simulink model "Simulink_IEEE_39_two_DSR"  (R2021b)
settings: Solver=ode23  StartTime=0.0  StopTime=60  MaxStep=0.2  MinStep=0.0001  RelTol=1e-3  EnableMultiTasking=on
values from neighbouring files (symbols this model uses):
  A = 80    [Monte_Carlo_Simulation.m]
  AC = 0.01    [Monte_Carlo_Simulation.m]
  D = 125    [Monte_Carlo_Simulation.m]
  dP = -300    [Monte_Carlo_Simulation.m]
  FHP = 0.8    [Monte_Carlo_Simulation.m]
  H = 300    [Monte_Carlo_Simulation.m]
  N = 6000/1000    (= 6)    [Monte_Carlo_Simulation.m]
  Pa = DSR_max * rand(1,1)    [Monte_Carlo_Simulation.m]
  Pb = B_max * rand(1,1)    [Monte_Carlo_Simulation.m]
  R = 0.002* ones(gen_num)    [Monte_Carlo_Simulation.m]
  Re = PFR_max .* rand(1,10)    [Monte_Carlo_Simulation.m]
  Ta = 5    [Monte_Carlo_Simulation.m]
  TB = 0.5    [Monte_Carlo_Simulation.m]
  Tc = 0.27    [Monte_Carlo_Simulation.m]
  TCH = 0.6 * ones(10)    [Monte_Carlo_Simulation.m]
  TG = [0.3;0.4;0.5;0.3;0.4;0.5;0.5;0.3;0.4;0.5]*40    [Monte_Carlo_Simulation.m]
  TRH = 5    [Monte_Carlo_Simulation.m]
settings Model: Creator=however  LastModifiedBy=e0546041
settings SolverCC: AlgebraicLoopSolver=TrustRegion
settings DataIOCC: LimitDataPoints=on  SaveFormat=Array  SignalLoggingSaveFormat=ModelDataLogs  ReturnWorkspaceOutputs=off
settings OptimizationCC: ExpressionDepthLimit=2147483647  LifeSpan=inf
settings DebuggingCC: UnderspecifiedInitializationDetection=Classic  MergeDetectMultiDrivingBlocksExec=none  SolverPrmCheckMsg=warning  FcnCallInpInsideContextMsg=warning  StateNameClashWarn=warning  PregeneratedLibrarySubsystemCodeDiagnostic=none  SFUnexpectedBacktrackingDiag=warning  SFNoUnconditionalDefaultTransitionDiag=warning  SFExecutionAtInitializationDiag=none  SFMachineParentedDataDiag=warning  ArithmeticOperatorsInVariantConditions=warning
settings HardwareCC: ProdBitPerPointer=32  ProdBitPerSizeT=32  ProdBitPerPtrDiffT=32  ProdLargestAtomicFloat=None  ProdIntDivRoundTo=Undefined  ProdEndianess=Unspecified  ProdWordSize=32  ProdHWDeviceType=32-bit Generic
settings ModelReferenceCC: PropagateSignalLabelsOutOfModel=off
settings SFSimCC: SimUseLocalCustomCode=off  CustomCodeUndefinedFunction=UseInterfaceOnly
settings RTWCC: RTWUseLocalCustomCode=off
settings CodeAppCC: StateflowObjectComments=on
settings GRTTargetCC: TargetLangStandard=C89/C90 (ANSI)  CombineOutputUpdateFcns=off  GRTInterface=on
settings ConfigComp: CovMetricSettings=dw  CovSaveCumulativeToWorkspaceVar=on  CovSaveSingleToWorkspaceVar=on  CovExternalEMLEnable=off

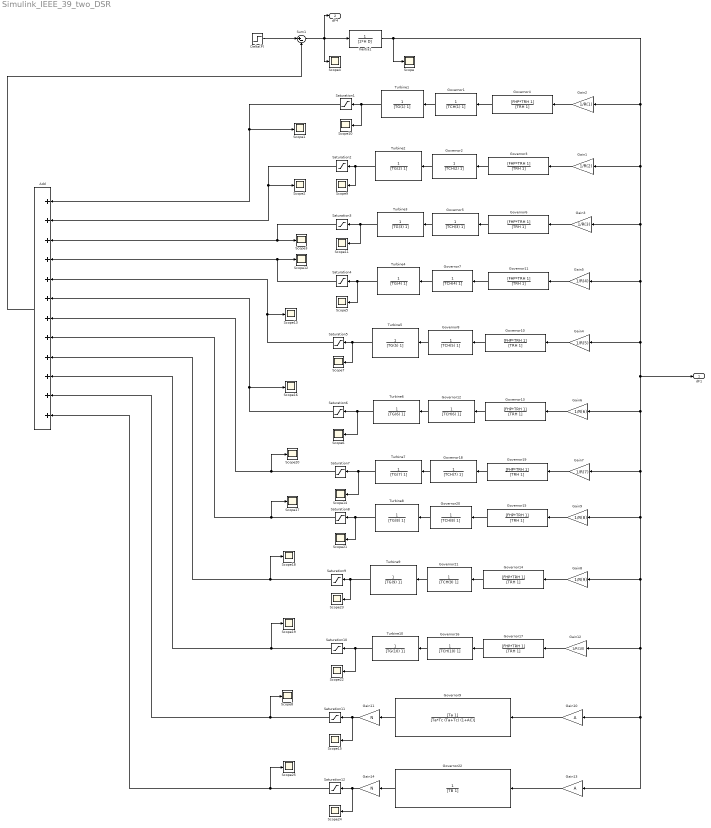
== system Simulink_IEEE_39_two_DSR ==
  Add : Sum  Inputs=++++++++++++
  Delta(P) : Step  Time=0  After=dP  SampleTime=0
  Gain1 : Gain  Gain=1/R(2)
  Gain10 : Gain  Gain=A
  Gain11 : Gain  Gain=N
  Gain12 : Gain  Gain=1/R(10)
  Gain13 : Gain  Gain=A
  Gain14 : Gain  Gain=N
  Gain2 : Gain  Gain=1/R(1)
  Gain3 : Gain  Gain=1/R(3)
  Gain4 : Gain  Gain=1/R(5)
  Gain5 : Gain  Gain=1/R(4)
  Gain6 : Gain  Gain=1/R(6)
  Gain7 : Gain  Gain=1/R(7)
  Gain8 : Gain  Gain=1/R(9)
  Gain9 : Gain  Gain=1/R(8)
  Governor1 : TransferFcn  Denominator=[TCH(1) 1]
  Governor{3..4,6,10..11,13..15,17,19} (10 alike) : TransferFcn  Numerator=[FHP*TRH 1]  Denominator=[TRH 1]
  Governor12 : TransferFcn  Denominator=[TCH(6) 1]
  Governor16 : TransferFcn  Denominator=[TCH(10) 1]
  Governor18 : TransferFcn  Denominator=[TCH(7) 1]
  Governor2 : TransferFcn  Denominator=[TCH(2) 1]
  Governor20 : TransferFcn  Denominator=[TCH(8) 1]
  Governor21 : TransferFcn  Denominator=[TCH(9) 1]
  Governor22 : TransferFcn  Denominator=[TB 1]
  Governor5 : TransferFcn  Denominator=[TCH(3) 1]
  Governor7 : TransferFcn  Denominator=[TCH(4) 1]
  Governor8 : TransferFcn  Denominator=[TCH(5) 1]
  Governor9 : TransferFcn  Numerator=[Ta 1]  Denominator=[Ta*Tc (Ta+Tc) (1+AC)]
  Inertia1 : TransferFcn  Denominator=[2*H D]
  Saturation1 : Saturate  UpperLimit=Re(1)  LowerLimit=-Re(1)
  Saturation10 : Saturate  UpperLimit=Re(10)  LowerLimit=-Re(10)
  Saturation11 : Saturate  UpperLimit=Pa(1)  LowerLimit=-Pa(1)
  Saturation12 : Saturate  UpperLimit=Pb  LowerLimit=-Pb
  Saturation2 : Saturate  UpperLimit=Re(2)  LowerLimit=-Re(2)
  Saturation3 : Saturate  UpperLimit=Re(3)  LowerLimit=-Re(3)
  Saturation4 : Saturate  UpperLimit=Re(4)  LowerLimit=-Re(4)
  Saturation5 : Saturate  UpperLimit=Re(5)  LowerLimit=-Re(5)
  Saturation6 : Saturate  UpperLimit=Re(6)  LowerLimit=-Re(6)
  Saturation7 : Saturate  UpperLimit=Re(7)  LowerLimit=-Re(7)
  Saturation8 : Saturate  UpperLimit=Re(8)  LowerLimit=-Re(8)
  Saturation9 : Saturate  UpperLimit=Re(9)  LowerLimit=-Re(9)
  Scope{,1..25} (26 alike) : Scope
  Sum1 : Sum  Inputs=|+-
  Turbine1 : TransferFcn  Denominator=[TG(1) 1]
  Turbine10 : TransferFcn  Denominator=[TG(10) 1]
  Turbine2 : TransferFcn  Denominator=[TG(2) 1]
  Turbine3 : TransferFcn  Denominator=[TG(3) 1]
  Turbine4 : TransferFcn  Denominator=[TG(4) 1]
  Turbine5 : TransferFcn  Denominator=[TG(5) 1]
  Turbine6 : TransferFcn  Denominator=[TG(6) 1]
  Turbine7 : TransferFcn  Denominator=[TG(7) 1]
  Turbine8 : TransferFcn  Denominator=[TG(8) 1]
  Turbine9 : TransferFcn  Denominator=[TG(9) 1]
  dF1 : Outport  VectorParamsAs1DForOutWhenUnconnected=off
  dF4 : Outport  Port=2  VectorParamsAs1DForOutWhenUnconnected=off
  wires:
  Governor1/1 -> Turbine1/1
  Governor4/1 -> Governor1/1
  Turbine1/1 -> Scope10/1, Saturation1/1
  Delta(P)/1 -> Sum1/1
  Governor3/1 -> Governor2/1
  Turbine2/1 -> Scope9/1, Saturation2/1
  Governor2/1 -> Turbine2/1
  Governor5/1 -> Turbine3/1
  Turbine3/1 -> Scope11/1, Saturation3/1
  Governor6/1 -> Governor5/1
  Saturation1/1 -> Scope1/1, Add/1
  Saturation2/1 -> Scope2/1, Add/2
  Add/1 -> Sum1/2
  Gain2/1 -> Governor4/1
  Gain1/1 -> Governor3/1
  Gain3/1 -> Governor6/1
  Saturation3/1 -> Scope3/1, Add/3
  Gain10/1 -> Governor9/1
  Governor9/1 -> Gain11/1
  Gain11/1 -> Scope15/1, Saturation11/1
  Saturation11/1 -> Scope8/1, Add/11
  Gain5/1 -> Governor11/1
  Saturation4/1 -> Add/4, Scope12/1
  Turbine4/1 -> Scope5/1, Saturation4/1
  Saturation5/1 -> Scope13/1, Add/5
  Governor12/1 -> Turbine6/1
  Gain4/1 -> Governor10/1
  Gain6/1 -> Governor13/1
  Governor11/1 -> Governor7/1
  Governor10/1 -> Governor8/1
  Turbine5/1 -> Scope7/1, Saturation5/1
  Saturation6/1 -> Scope16/1, Add/6
  Governor13/1 -> Governor12/1
  Turbine6/1 -> Scope6/1, Saturation6/1
  Governor8/1 -> Turbine5/1
  Governor7/1 -> Turbine4/1
  Saturation8/1 -> Add/8, Scope17/1
  Governor17/1 -> Governor16/1
  Saturation10/1 -> Scope19/1, Add/10
  Turbine8/1 -> Scope21/1, Saturation8/1
  Turbine9/1 -> Scope23/1, Saturation9/1
  Governor14/1 -> Governor21/1
  Governor15/1 -> Governor20/1
  Saturation9/1 -> Scope18/1, Add/9
  Gain8/1 -> Governor14/1
  Governor16/1 -> Turbine10/1
  Gain12/1 -> Governor17/1
  Gain9/1 -> Governor15/1
  Saturation7/1 -> Add/7, Scope20/1
  Turbine7/1 -> Scope14/1, Saturation7/1
  Gain7/1 -> Governor19/1
  Governor19/1 -> Governor18/1
  Governor18/1 -> Turbine7/1
  Turbine10/1 -> Scope22/1, Saturation10/1
  Governor20/1 -> Turbine8/1
  Governor21/1 -> Turbine9/1
  Inertia1/1 -> dF1/1, Gain6/1, Gain9/1, Gain8/1, Gain13/1, Gain10/1, Gain12/1, Gain7/1, Gain4/1, Gain5/1, Gain3/1, Gain1/1, Gain2/1, Scope/1
  Saturation12/1 -> Add/12, Scope25/1
  Gain13/1 -> Governor22/1
  Governor22/1 -> Gain14/1
  Gain14/1 -> Scope24/1, Saturation12/1
  Sum1/1 -> dF4/1, Scope4/1, Inertia1/1
